simulink model "lab11_test2"  (R2024a)
settings: Solver=VariableStepAuto  StartTime=0.0  StopTime=10.0  RelTol=1e-3
values from neighbouring files (symbols this model uses):
  m = m + 1    (= 2)    [lab5.m]
undefined symbols (not defined in the file or in its folder): n
libraries: simulink x2
settings Model: Creator=QQshnik  LastModifiedBy=QQshnik

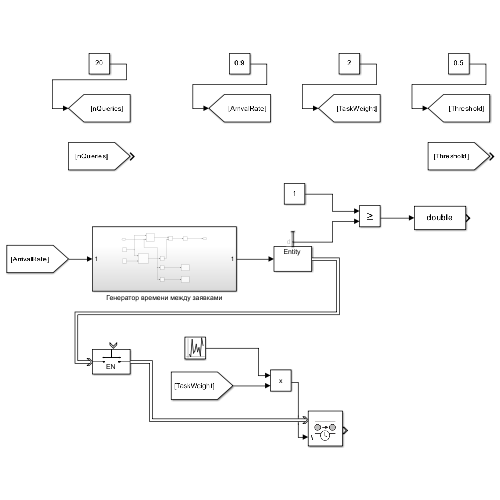
[thumbnail: Simulink's stored preview of the top-level diagram]
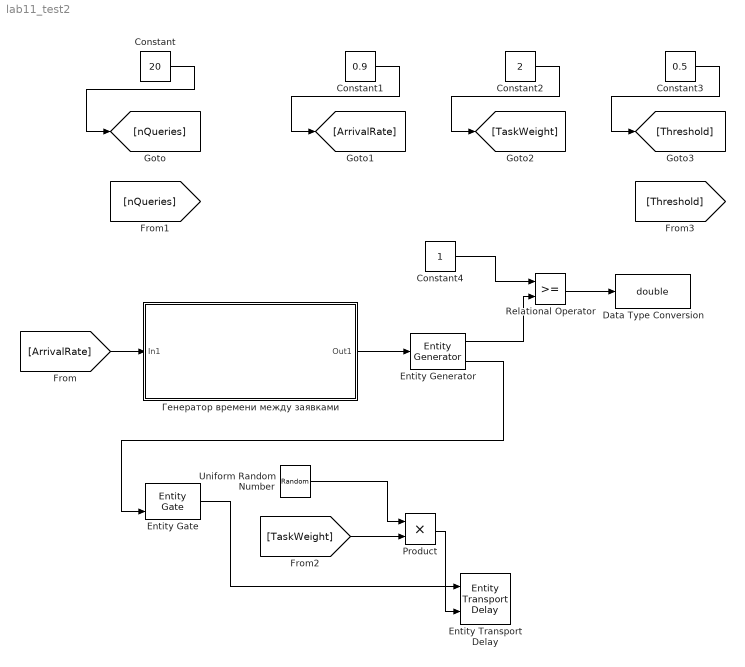
== system lab11_test2 ==
  Constant : Constant  Value=20
  Constant1 : Constant  Value=0.9
  Constant2 : Constant  Value=2
  Constant3 : Constant  Value=0.5
  Constant4 : Constant
  Data Type Conversion : DataTypeConversion  OutDataTypeStr=double  SaturateOnIntegerOverflow=off  RndMeth=Floor
  Entity Transport Delay : EntityTransportDelay  InputPortMessageModes=m,n  OutputPortMessageModes=m
  Entity Gate : EntityGate  InputPortMessageModes=m,m  OutputPortMessageModes=m
  Entity Generator : EntityGenerator  OutputPortMessageModes=n,m  TimeSource=Signal port  NumberEntitiesDeparted=on  EntityType=Structured  EntityTypeName=Entity
      settings: InputPortMap=u1  OutputPortMap=o0,o3
  Product : Product
  Relational Operator : RelationalOperator  OutDataTypeStr=boolean  RndMeth=Simplest  InputSameDT=off
  Uniform Random Number : UniformRandomNumber  SampleTime=0.1
  Генератор времени между заявками : Subsystem
  wires:
  Constant/1 -> [nQueries]
  Constant1/1 -> [ArrivalRate]
  Constant2/1 -> [TaskWeight]
  Constant3/1 -> [Threshold]
  [ArrivalRate] -> Генератор времени между заявками/1(In1)
  Генератор времени между заявками/1(Out1) -> Entity Generator/1
  Relational Operator/1 -> Data Type Conversion/1
  Constant4/1 -> Relational Operator/1
  Entity Generator/1 -> Relational Operator/2
  Entity Generator/2 -> Entity Gate/2
  Uniform Random Number/1 -> Product/1
  Product/1 -> Entity Transport Delay/2
  [TaskWeight] -> Product/2
  Entity Gate/1 -> Entity Transport Delay/1

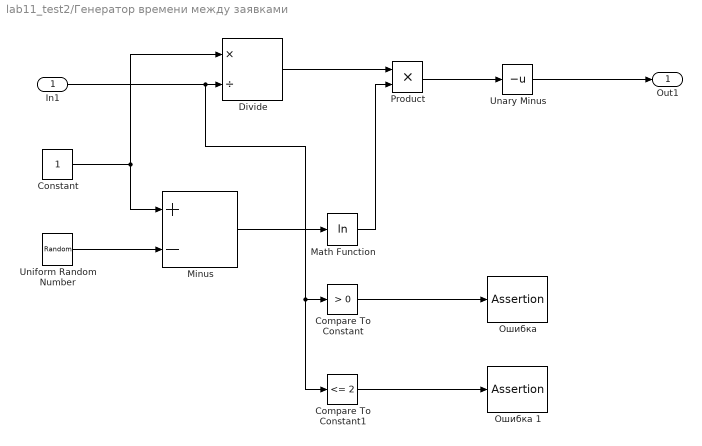
== system lab11_test2/Генератор времени между заявками ==
  In1 : Inport
  Compare To Constant : simulink/Logic and Bit Operations/Compare To Constant  relop=>  const=0  OutDataTypeStr=boolean
  Compare To Constant1 : simulink/Logic and Bit Operations/Compare To Constant  relop=<=  const=2  OutDataTypeStr=boolean
  Constant : Constant
  Divide : Product  Inputs=*/
  Math Function : Math  Operator=log
  Minus : Sum  Inputs=+-
  Product : Product
  Unary Minus : UnaryMinus
  Uniform Random Number : UniformRandomNumber  SampleTime=0.1
  Ошибка : Assertion
  Ошибка 1 : Assertion
  Out1 : Outport
  wires:
  Constant/1 -> Divide/1, Minus/1
  In1/1 -> Compare To Constant1/1, Compare To Constant/1, Divide/2
  Math Function/1 -> Product/2
  Uniform Random Number/1 -> Minus/2
  Minus/1 -> Math Function/1
  Compare To Constant/1 -> Ошибка/1
  Divide/1 -> Product/1
  Compare To Constant1/1 -> Ошибка 1/1
  Product/1 -> Unary Minus/1
  Unary Minus/1 -> Out1/1
